simulink model "stm32_multitasking_gettingstarted_J"  (R2022b)
settings: Solver=FixedStepAuto  StartTime=0.0  StopTime=10.0  RelTol=1e-3  EnableMultiTasking=on
libraries: stm32f4xxblockslib x2, simulink x1
settings Model: Creator=The MathWorks, Inc.  LastModifiedBy=siegeljb
settings SolverCC: AutoInsertRateTranBlk=on
settings OptimizationCC: EnhancedBackFolding=on  PassReuseOutputArgsAs=Individual arguments  ZeroExternalMemoryAtStartup=off  ZeroInternalMemoryAtStartup=off  MaxStackSize=64  OptimizeBlockOrder=speed  DifferentSizesBufferReuse=on  OptimizationCustomize=off  EfficientTunableParamExpr=on
settings DebuggingCC: ParameterTunabilityLossMsg=error  UnconnectedInputMsg=warning  UnconnectedOutputMsg=warning  UnconnectedLineMsg=warning
settings HardwareCC: ProdBitPerPointer=32  ProdBitPerSizeT=32  ProdBitPerPtrDiffT=32  ProdLargestAtomicInteger=Long  ProdLargestAtomicFloat=Double  ProdWordSize=32  ProdLongLongMode=on  ProdHWDeviceType=ARM Compatible->ARM Cortex
settings ModelReferenceCC: EnableRefExpFcnMdlSchedulingChecks=on
settings SFSimCC: MATLABDynamicMemAlloc=off
settings RTWCC: Description=Embedded Coder  SystemTargetFile=ert.tlc  HardwareBoard=STM32F4xx Based  TLCOptions=-aInlineSetEventsForThisBaseRateFcn=TLC_FALSE -aSuppressMultiTaskScheduler=TLC_FALSE -aRateBasedStepFcn=1  TemplateMakefile=ert_default_tmf  Toolchain=GNU Tools for ARM Embedded Processors  DLArmComputeVersion=19.05
settings CodeAppCC: ForceParamTrailComments=on  IgnoreCustomStorageClasses=off  OperatorAnnotations=on  SimulinkDataObjDesc=on  SFDataObjDesc=on  InsertBlockDesc=on
settings ERTTargetCC: CodeReplacementLibrary=ARM Cortex-M  ExtModeTransport=3  ExtModeStaticAlloc=on  ExtModeStaticAllocSize=8000  ExtModeMexFile=ext_xcp  ExtModeIntrfLevel=Level2 - Open

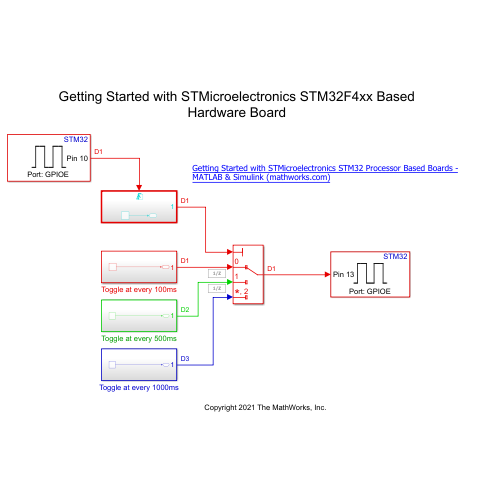
[thumbnail: Simulink's stored preview of the top-level diagram]
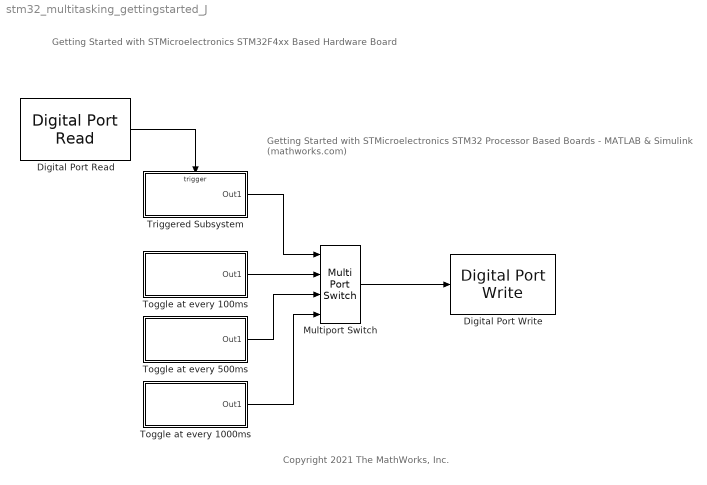
== system stm32_multitasking_gettingstarted_J ==
  note: Getting Started with STMicroelectronics STM32 Processor Based Boards - MATLAB & Simulink (mathworks.com)
  note: Getting Started with STMicroelectronics STM32F4xx Based Hardware Board
  note: Copyright 2021 The MathWorks, Inc.
  Digital Port Read : stm32f4xxblockslib/Digital Port Read  PortName=GPIOE  PinNumber=10  ReadOperation=on  IOAsArray=off  SampleTime=-1  EnableSimPort=off
  Digital Port Write : stm32f4xxblockslib/Digital Port Write  PortName=GPIOE  PinNumber=13  ReadOperation=off  IOAsArray=off  EnableSimPort=off
  Multiport Switch : MultiPortSwitch  DataPortOrder=Zero-based contiguous  zeroidx=on  SaturateOnIntegerOverflow=off  InputSameDT=off
  Toggle at every 1000ms : Subsystem
  Toggle at every 100ms : Subsystem
  Toggle at every 500ms : Subsystem
  Triggered Subsystem : Subsystem  TreatAsAtomicUnit=on
  wires:
  Digital Port Read/1 -> Triggered Subsystem/Trigger
  Toggle at every 1000ms/1(Out1) -> Multiport Switch/4
  Triggered Subsystem/1(Out1) -> Multiport Switch/1
  Toggle at every 500ms/1(Out1) -> Multiport Switch/3
  Toggle at every 100ms/1(Out1) -> Multiport Switch/2
  Multiport Switch/1 -> Digital Port Write/1

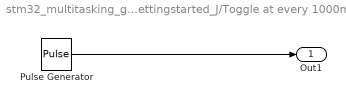
== system stm32_multitasking_gettingstarted_J/Toggle at every 1000ms ==
  Pulse Generator : DiscretePulseGenerator
  Out1 : Outport
  wires:
  Pulse Generator/1 -> Out1/1

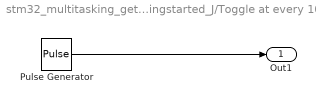
== system stm32_multitasking_gettingstarted_J/Toggle at every 100ms ==
  Pulse Generator : DiscretePulseGenerator  SampleTime=0.1
  Out1 : Outport
  wires:
  Pulse Generator/1 -> Out1/1

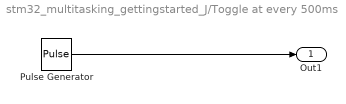
== system stm32_multitasking_gettingstarted_J/Toggle at every 500ms ==
  Pulse Generator : DiscretePulseGenerator  SampleTime=0.5
  Out1 : Outport
  wires:
  Pulse Generator/1 -> Out1/1

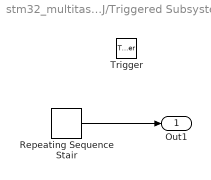
== system stm32_multitasking_gettingstarted_J/Triggered Subsystem ==
  Trigger : TriggerPort  VariantControl=(inherit)
  Repeating Sequence Stair : simulink/Sources/Repeating Sequence Stair  OutValues=[1 2 0]  tsamp=-1  OutMin=[]  OutMax=[]  OutDataTypeStr=double  OutputDataTypeScalingMode=double  OutDataType=fixdt(0,8)  ConRadixGroup=Best Precision: Vector-wise  OutScaling=2^-12
  Out1 : Outport
  wires:
  Repeating Sequence Stair/1 -> Out1/1
